simulink model "boost_converter"  (R2021b)
settings: Solver=ode45  StartTime=0.0  StopTime=0.05  RelTol=1e-3
libraries: spsSeriesRLCBranchLib x3, spsMultimeterLib x2, spsDCVoltageSourceLib x1, spsDiodeLib x1, spsMosfetLib x1, spsVoltageMeasurementLib x1, spspowerguiLib x1
settings Model: Creator=goyal  LastModifiedBy=Asus

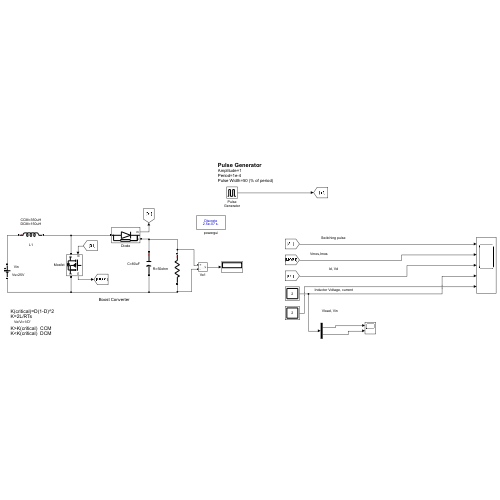
[thumbnail: Simulink's stored preview of the top-level diagram]
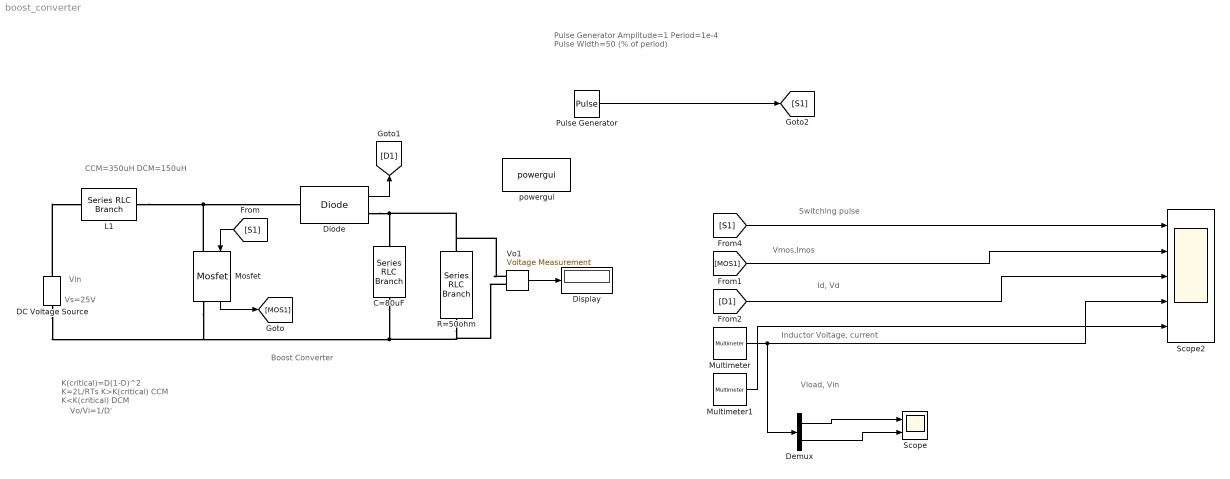
== system boost_converter ==
  note: Vo/Vi=1/D'
  note: Boost Converter
  note: K(critical)=D(1-D)^2
      | K=2L/RTs
      |
      | K>K(critical) CCM
      | K<K(critical) DCM
  note: Pulse Generator
      | Amplitude=1
      | Period=1e-4
      | Pulse Width=50 (% of period)
  note: CCM=350uH
      | DCM=150uH
  note: Vs=25V
  note: Vin
  note: Id, Vd
  note: Vmos,Imos
  note: Switching pulse
  note: Inductor Voltage, current
  note: Vload, Vin
  C=80uF : spsSeriesRLCBranchLib/Series RLC Branch  LConnTagsString=__new0  RConnTagsString=__new0  BranchType=C  Resistance=1  Inductance=1e-3  SetiL0=off  InitialCurrent=0  Capacitance=80e-6  Setx0=off  InitialVoltage=0  Measurements=None
  DC Voltage Source : spsDCVoltageSourceLib/DC Voltage Source  Amplitude=25  Measurements=Voltage
  Demux : Demux  Outputs=2
  Diode : spsDiodeLib/Diode  Ron=0.001  Lon=0  Vf=0.8  IC=0  UseSnubber=0  Rs=500  Cs=250e-9  Measurements=on
  Display : Display
  L1 : spsSeriesRLCBranchLib/Series RLC Branch  LConnTagsString=__new0  RConnTagsString=__new0  BranchType=L  Resistance=1  Inductance=350e-6  SetiL0=off  InitialCurrent=0  Capacitance=1e-6  Setx0=off  InitialVoltage=0  Measurements=Branch voltage and current
  Mosfet : spsMosfetLib/Mosfet  Ron=0.1  Lon=0  Rd=0.01  Vfd=0  IC=0  Rs=1e5  Cs=inf  Measurements=on
  Multimeter : spsMultimeterLib/Multimeter  PhasorSimulation=off  OutputType=Complex  sel=[1 4]  L=4  Gain=[1 1]  yselected={'Ub: L1','Ib: L1'};  PSBOutputType=1  PSBequivalent=0  AxesSetting=[0,0.1,-100,100]  Display=0  SavedBlockNames=-11
  Multimeter1 : spsMultimeterLib/Multimeter  PhasorSimulation=off  OutputType=Complex  sel=[3 2]  L=4  Gain=[1 1]  yselected={'Usrc: DC Voltage Source','Ub: R=50ohm'};  PSBOutputType=1  PSBequivalent=0  AxesSetting=[0,0.1,-100,100]  Display=0  SavedBlockNames=-11
  Pulse Generator : DiscretePulseGenerator  PulseType=Time based  Period=1e-4  PulseWidth=50
  R=50ohm : spsSeriesRLCBranchLib/Series RLC Branch  LConnTagsString=__new0  RConnTagsString=__new0  BranchType=R  Resistance=50  Inductance=1e-3  SetiL0=off  InitialCurrent=0  Capacitance=1e-6  Setx0=off  InitialVoltage=0  Measurements=Branch voltage
  Scope : Scope  NumInputPorts=2
  Scope2 : Scope  NumInputPorts=5
  Vo1 : spsVoltageMeasurementLib/Voltage Measurement  PhasorSimulation=off  OutputType=Complex  PSBequivalent=0
  powergui : spspowerguiLib/powergui  Priority=1  SimulationMode=Discrete  SampleTime=2.5e-7  frequency=60  Iterations=50  frequencyindice=0  Pbase=100e6  ErrMax=1e-4  UnitsV=kV  UnitsW=MW  buscounter=0  FunctionMessages=off  echomessages=off  EnableUseOfTLC=off  CurrentSourceSwitches=off  DisableSnubberDevices=off  DisableRonSwitches=off  DisableVfSwitches=off  DisplayEquations=off  AutomaticDiscreteSolvers=off  SolverType=Tustin/Backward Euler (TBE)  Interpol=off  ExternalGateDelay=off  methode=off  Ts=100  x0status=blocks  SPID=on  SwTol=0  HookPort=off  NonlinearTolerance=1e-4  nMaxIteration=100  ContinueOnMaxIteration=off  RestoreLinks=warning  ResistiveCurrentMeasurement=off  Frange=[0:2:500]  Ylog=off  Xlog=on  ShowGrid=off  save=off  variable=ZData  structure=0  ZoomFFT=off  StartTime=0.0  cycles=1  DisplayStyle=1  fundamental=60  FreqAxis=off  MaxFrequency=1000  frequencyindicesteady=1  RmsSteady=1  display=off
  wires:
  Vo1/1 -> Display/1
  Multimeter/1 -> Demux/1, Scope2/4
  Mosfet/1 -> [MOS1]
  Pulse Generator/1 -> [S1]
  [S1] -> Mosfet/1
  [MOS1] -> Scope2/2
  Multimeter1/1 -> Scope2/5
  Diode/1 -> [D1]
  [S1] -> Scope2/1
  [D1] -> Scope2/3
  Demux/1 -> Scope/1
  Demux/2 -> Scope/2
  connections:
  Vo1/LConn1 -- R=50ohm/LConn1 -- Diode/RConn1 -- C=80uF/LConn1
  C=80uF/RConn1 -- Mosfet/RConn1 -- DC Voltage Source/LConn1 -- Vo1/LConn2 -- R=50ohm/RConn1
  Mosfet/LConn1 -- Diode/LConn1 -- L1/RConn1
  DC Voltage Source/RConn1 -- L1/LConn1
